simulink model "OMAP_ver_MIL10"  (R2018b)
settings: Solver=FixedStepDiscrete  StartTime=0.0  StopTime=10.0  FixedStep=0.01  RelTol=1e-3
undefined symbols (not defined in the file or in its folder): OMAP_Switch_EMS, OMAP_Switch_EPS, OMAP_Switch_ESC, OMAP_Switch_IC, OMAP_Switch_OTHER, TH_HMIClb_tiDgrdIconWarnHiDurT_C, TH_HMIClb_tiDgrdIconWarnLoDurT_C, TH_HMIClb_tiDgrdVocWarnDurT_C, TH_HMIClb_tiHndOffTxtWarnT_C, TH_HMIClb_tiHndOffVocWarnT_C, TH_HMIClb_tiSWALimFlgDetT_C, TH_HMIClb_tiTxtLimT_C
libraries: simulink x118
(part 7 of 9)

== system OMAP_ver_MIL10/OMAP_Module/ACCS_Direct/ACCS_Define/Human_Machine_Interface(ACC_HMI)/Text_PopUp/ACC_ON ==
  In1 : Inport
  In2 : Inport  Port=2
  ACCICA_Flag : Inport  Port=3
  Chart : Stateflow chart  TreatAsAtomicUnit=on
  Compare To Constant{1..2,6,9} (4 alike) : simulink/Logic and Bit Operations/Compare To Constant  relop===  const=1  OutDataTypeStr=boolean
  Compare To Constant10 : simulink/Logic and Bit Operations/Compare To Constant  relop=~=  const=1  OutDataTypeStr=boolean
  Compare To Constant11 : simulink/Logic and Bit Operations/Compare To Constant  relop=~=  const=15  OutDataTypeStr=boolean
  Compare To Constant14 : simulink/Logic and Bit Operations/Compare To Constant  relop===  const=3  OutDataTypeStr=boolean
  Compare To Constant3 : simulink/Logic and Bit Operations/Compare To Constant  relop===  const=2  OutDataTypeStr=boolean
  Compare To Constant4 : simulink/Logic and Bit Operations/Compare To Constant  relop=~=  const=1  OutDataTypeStr=boolean
  Compare To Constant5 : simulink/Logic and Bit Operations/Compare To Constant  relop=~=  const=0  OutDataTypeStr=boolean
  Compare To Constant7 : simulink/Logic and Bit Operations/Compare To Constant  relop===  const=0  OutDataTypeStr=boolean
  Compare To Constant8 : simulink/Logic and Bit Operations/Compare To Constant  relop===  const=0  OutDataTypeStr=boolean
  Logical Operator : Logic  Inputs=3  AllPortsSameDT=off  OutDataTypeStr=boolean
  Logical Operator1 : Logic  AllPortsSameDT=off  OutDataTypeStr=boolean
  Logical Operator2 : Logic  AllPortsSameDT=off  OutDataTypeStr=boolean
  Logical Operator3 : Logic  AllPortsSameDT=off  OutDataTypeStr=boolean
  Logical Operator4 : Logic  Operator=OR  AllPortsSameDT=off  OutDataTypeStr=boolean
  Logical Operator5 : Logic  Inputs=3  AllPortsSameDT=off  OutDataTypeStr=boolean
  Logical Operator9 : Logic  Operator=OR  AllPortsSameDT=off  OutDataTypeStr=boolean
  Unit Delay : UnitDelay  SampleTime=-1
  Unit Delay1 : UnitDelay  SampleTime=-1
  Unit Delay2 : UnitDelay  SampleTime=-1
  Out1 : Outport
  wires:
  Compare To Constant14/1 -> Logical Operator9/2
  Compare To Constant1/1 -> Logical Operator/1
  Logical Operator/1 -> Chart/1(data)
  Logical Operator9/1 -> Logical Operator/2
  Unit Delay/1 -> Compare To Constant1/1
  Compare To Constant3/1 -> Logical Operator9/1
  Chart/1(Value) -> Out1/1
  In2/1 -> Compare To Constant4/1, Unit Delay1/1
  Unit Delay1/1 -> Compare To Constant2/1
  Compare To Constant2/1 -> Logical Operator1/1
  Compare To Constant4/1 -> Logical Operator1/2
  Logical Operator4/1 -> Chart/2(data1)
  In1/1 -> Compare To Constant11/1, Compare To Constant10/1, Compare To Constant5/1, Compare To Constant14/1, Compare To Constant3/1, Unit Delay/1
  Logical Operator5/1 -> Logical Operator2/2
  ACCICA_Flag/1 -> Compare To Constant8/1, Compare To Constant9/1, Compare To Constant7/1, Unit Delay2/1
  Unit Delay2/1 -> Compare To Constant6/1
  Compare To Constant6/1 -> Logical Operator3/1
  Compare To Constant7/1 -> Logical Operator3/2
  Logical Operator3/1 -> Logical Operator2/1
  Logical Operator2/1 -> Chart/3(data2)
  Compare To Constant8/1 -> Logical Operator/3
  Logical Operator1/1 -> Logical Operator4/2
  Compare To Constant9/1 -> Logical Operator4/1
  Compare To Constant5/1 -> Logical Operator5/1
  Compare To Constant10/1 -> Logical Operator5/2
  Compare To Constant11/1 -> Logical Operator5/3

== system OMAP_ver_MIL10/OMAP_Module/ACCS_Direct/ACCS_Define/Human_Machine_Interface(ACC_HMI)/Text_PopUp/ACC_go_request ==
  In1 : Inport
  Compare To Constant1 : simulink/Logic and Bit Operations/Compare To Constant  relop===  const=1  OutDataTypeStr=boolean
  <GoRequest> : Outport
  wires:
  In1/1 -> Compare To Constant1/1
  Compare To Constant1/1 -> <GoRequest>/1

== system OMAP_ver_MIL10/OMAP_Module/ACCS_Direct/ACCS_Define/Human_Machine_Interface(ACC_HMI)/Text_PopUp/Please_Take_Over_the_Car ==
  In1 : Inport
  Chart1 : Stateflow chart  TreatAsAtomicUnit=on
  Compare To Constant1 : simulink/Logic and Bit Operations/Compare To Constant  relop===  const=6  OutDataTypeStr=boolean
  Compare To Constant18 : simulink/Logic and Bit Operations/Compare To Constant  relop===  const=6  OutDataTypeStr=boolean
  Compare To Constant19 : simulink/Logic and Bit Operations/Compare To Constant  relop===  const=4  OutDataTypeStr=boolean
  Compare To Constant2 : simulink/Logic and Bit Operations/Compare To Constant  relop=~=  const=6  OutDataTypeStr=boolean
  Logical Operator1 : Logic  AllPortsSameDT=off  OutDataTypeStr=boolean
  Logical Operator7 : Logic  AllPortsSameDT=off  OutDataTypeStr=boolean
  Unit Delay1 : UnitDelay  SampleTime=-1
  Unit Delay2 : UnitDelay  SampleTime=-1
  Out1 : Outport
  wires:
  Logical Operator7/1 -> Chart1/1(IN)
  Compare To Constant18/1 -> Logical Operator7/2
  Unit Delay2/1 -> Compare To Constant19/1
  Compare To Constant19/1 -> Logical Operator7/1
  Chart1/1(Value) -> Out1/1
  Unit Delay1/1 -> Compare To Constant1/1
  Compare To Constant1/1 -> Logical Operator1/1
  Compare To Constant2/1 -> Logical Operator1/2
  Logical Operator1/1 -> Chart1/2(OUT)
  In1/1 -> Unit Delay1/1, Compare To Constant2/1, Compare To Constant18/1, Unit Delay2/1

== system OMAP_ver_MIL10/OMAP_Module/ACCS_Direct/ACCS_Define/Human_Machine_Interface(ACC_HMI)/Text_PopUp/Please_Take_Over_the_Car_immediataly ==
  ESC_DecTar : Inport
  BRAKE_RELEASED_FAILSAFE1 : Constant  Value=0  OutDataTypeStr=boolean
  Chart1 : Stateflow chart  TreatAsAtomicUnit=on
  Out1 : Outport
  wires:
  Chart1/1(Value) -> Out1/1
  ESC_DecTar/1 -> Chart1/1(ESC_DecTar)
  BRAKE_RELEASED_FAILSAFE1/1 -> Chart1/2(BRAKE_RELEASED_FAILSAFE)

== system OMAP_ver_MIL10/OMAP_Module/ICA_Direct_G59/ICA_Define/Subsystem1/Dspl/DsplPrcs ==
  DsplPrcs_stStWhlHld : Inport
  DsplPrcs_stTkOvStChk : Inport  Port=2
  DsplPrcs_facmL0Ql : Inport  Port=3
  DsplPrcs_facmR0Ql : Inport  Port=4
  DsplPrcs_facmL0Type : Inport  Port=5
  DsplPrcs_facmR0Type : Inport  Port=6
  DsplPrcs_stTHState : Inport  Port=7
  DsplPrcs_bsFromFMCMsg : Inport  Port=8
  DsplPrcs_stTHFKeyState : Inport  Port=9
  DsplPrcs_stVehSty : Inport  Port=10
  DsplPrcs_tfAddVocCmd : Inport  Port=11
  DsplPrcs_stSWALimFlg : Inport  Port=12
  DsplPrcs_dHndOffTxtWarnnum : Inport  Port=13
  DsplPrcs_dDgrdVocWarnDurnum : Inport  Port=14
  DsplPrcs_dHndOffVocWarnnum : Inport  Port=15
  DsplPrcs_dTxtLimnum : Inport  Port=16
  DsplPrcs_dDgrdIconWarnHiDurnum : Inport  Port=17
  DsplPrcs_dDgrdIconWarnLoDurnum : Inport  Port=18
  DsplPrcs_tiSWALimFlgDetnum : Inport  Port=19
  DsplPrcs_dDgrdIconWarnflag : Inport  Port=20
  Bus Creator1 : BusCreator  Inputs=4
  Bus Selector : BusSelector  OutputSignals=stLaneDspl,stL0DispType,stR0DispType
  Bus Selector1 : BusSelector  OutputSignals=ACC_State
  Data Type Conversion1 : DataTypeConversion  OutDataTypeStr=uint16
  Icon : Subsystem
  Lane : Subsystem
  Lane_old : Subsystem
  Manual Switch : ManualSwitch
  Txt : Subsystem
  Voc : Subsystem
  DsplPrcs_stTxtDspl : Outport
  DsplPrcs_stIconDspl : Outport  Port=2
  DsplPrcs_stLaneDspl : Outport  Port=3
  DsplPrcs_stL0DispType : Outport  Port=4
  DsplPrcs_stR0DispType : Outport  Port=5
  DsplPrcs_stVocDspl : Outport  Port=6
  DsplPrcs_bsMon : Outport  Port=7
  wires:
  DsplPrcs_stTHFKeyState/1 -> Txt/4(Txt_stTHFKeyState)
  Txt/1(Txt_stTxtDspl) -> DsplPrcs_stTxtDspl/1
  DsplPrcs_stTHState/1 -> Txt/6(Txt_stTHState), Lane_old/1(Lane_stTHState), Voc/2(Voc_stTHState), Lane/1(Lane_stTHState), Icon/1(Icon_stTHState)
  Icon/1(Icon_stIconDspl) -> Bus Creator1/2, DsplPrcs_stIconDspl/1  "ICA_status_icon"
  Lane/1(Lane_stLaneDspl) -> Bus Creator1/3, Bus Selector/1  "Vehicle_Lane_Display"
  Txt/2(Txt_bsMon) -> Bus Creator1/1  "ICA_HMI_Txt_Mon"
  Bus Creator1/1 -> DsplPrcs_bsMon/1
  DsplPrcs_stStWhlHld/1 -> Voc/1(Voc_stStWhlHld), Txt/1(Txt_stStWhlHld)
  DsplPrcs_dHndOffTxtWarnnum/1 -> Txt/5(Txt_dHndOffTxtWarnnum)
  Voc/1(Voc_stVocDspl) -> DsplPrcs_stVocDspl/1, Bus Creator1/4  "Hands_off_warning"
  DsplPrcs_dHndOffVocWarnnum/1 -> Voc/4(Voc_dHndOffVocWarnnum)
  DsplPrcs_dDgrdVocWarnDurnum/1 -> Voc/3(Voc_dDgrdVocWarnDurnum)
  DsplPrcs_bsFromFMCMsg/1 -> Txt/3(Txt_bsFromFMCMsg), Bus Selector1/1
  Data Type Conversion1/1 -> Icon/2(Icon_stACCState)
  Bus Selector1/1 -> Data Type Conversion1/1  "<ACC_State>"
  DsplPrcs_dTxtLimnum/1 -> Txt/7(Txt_dTxtLimnum)
  DsplPrcs_facmL0Ql/1 -> Lane_old/3(Lane_facmL0Ql), Lane/3(Lane_facmL0Ql)
  DsplPrcs_facmR0Ql/1 -> Lane_old/4(Lane_facmR0Ql), Lane/4(Lane_facmR0Ql)
  DsplPrcs_stVehSty/1 -> Lane/2(Lane_stVehSty), Lane_old/2(Lane_stVehSty), Voc/5(Voc_stVehSty), Txt/2(Txt_stVehSty)
  DsplPrcs_tfAddVocCmd/1 -> Voc/6(Voc_tfAddVocCmd)
  DsplPrcs_dDgrdIconWarnHiDurnum/1 -> Icon/3(Icon_dDgrdIconWarnHiDurnum)
  DsplPrcs_dDgrdIconWarnLoDurnum/1 -> Icon/4(Icon_dDgrdIconWarnLoDurnum)
  DsplPrcs_dDgrdIconWarnflag/1 -> Icon/5(Icon_dDgrdIconWarnflag)
  DsplPrcs_stSWALimFlg/1 -> Txt/8(Txt_stSWALimFlg)
  DsplPrcs_tiSWALimFlgDetnum/1 -> Txt/9(Txt_tiSWALimFlgDetnum)
  DsplPrcs_stTkOvStChk/1 -> Txt/10(Txt_stTkOvStChk)
  DsplPrcs_facmL0Type/1 -> Lane/5(Lane_facmL0Type)
  DsplPrcs_facmR0Type/1 -> Lane/6(Lane_facmR0Type)
  Bus Selector/1 -> Manual Switch/1  "<stLaneDspl>"
  Bus Selector/2 -> DsplPrcs_stL0DispType/1  "<stL0DispType>"
  Bus Selector/3 -> DsplPrcs_stR0DispType/1  "<stR0DispType>"
  Lane_old/1(Lane_stLaneDspl) -> Manual Switch/2
  Manual Switch/1 -> DsplPrcs_stLaneDspl/1

== system OMAP_ver_MIL10/OMAP_Module/ICA_Direct_G59/ICA_Define/Subsystem1/Dspl/TimePrcs ==
  TimePrcs_tiHndOffTxtWarnT_C : Inport
  TimePrcs_tiDgrdVocWarnDurT_C : Inport  Port=2
  TimePrcs_tiHndOffVocWarnT_C : Inport  Port=3
  TimePrcs_tiTxtLimT_C : Inport  Port=4
  TimePrcs_tiDgrdIconWarnHiDurT_C : Inport  Port=5
  TimePrcs_tiDgrdIconWarnLoDurT_C : Inport  Port=6
  TimePrcs_tiSWALimFlgDetT_C : Inport  Port=7
  TimePrcs_tiCalcPer_C : Inport  Port=8
  Divide{,1..6} (7 alike) : Product  Inputs=*/  OutDataTypeStr=uint16
  Switch : Switch  Criteria=u2 ~= 0  OutDataTypeStr=single
  constant : Constant  Value=0.01  OutDataTypeStr=single
  TimePrcs_dHndOffTxtWarnnum : Outport
  TimePrcs_dDgrdVocWarnDurnum : Outport  Port=2
  TimePrcs_dHndOffVocWarnnum : Outport  Port=3
  TimePrcs_dTxtLimnum : Outport  Port=4
  TimePrcs_dDgrdIconWarnHiDurnum : Outport  Port=5
  TimePrcs_dDgrdIconWarnLoDurnum : Outport  Port=6
  TimePrcs_tiSWALimFlgDetnum : Outport  Port=7
  wires:
  Divide/1 -> TimePrcs_dHndOffTxtWarnnum/1
  TimePrcs_tiCalcPer_C/1 -> Switch/1, Switch/2
  constant/1 -> Switch/3
  TimePrcs_tiHndOffTxtWarnT_C/1 -> Divide/1
  Switch/1 -> Divide5/2, Divide4/2, Divide3/2, Divide2/2, Divide1/2, Divide/2, Divide6/2
  TimePrcs_tiDgrdVocWarnDurT_C/1 -> Divide1/1
  TimePrcs_tiHndOffVocWarnT_C/1 -> Divide2/1
  TimePrcs_tiTxtLimT_C/1 -> Divide3/1
  Divide1/1 -> TimePrcs_dDgrdVocWarnDurnum/1
  Divide2/1 -> TimePrcs_dHndOffVocWarnnum/1
  Divide3/1 -> TimePrcs_dTxtLimnum/1
  TimePrcs_tiDgrdIconWarnHiDurT_C/1 -> Divide4/1
  Divide4/1 -> TimePrcs_dDgrdIconWarnHiDurnum/1
  TimePrcs_tiDgrdIconWarnLoDurT_C/1 -> Divide5/1
  Divide5/1 -> TimePrcs_dDgrdIconWarnLoDurnum/1
  Divide6/1 -> TimePrcs_tiSWALimFlgDetnum/1
  TimePrcs_tiSWALimFlgDetT_C/1 -> Divide6/1

== system OMAP_ver_MIL10/OMAP_Module/ICA_Direct_G59/ICA_Define/Subsystem1/Subsystem/Subsystem ==
  HiDurnum : Inport
  LoDurnum : Inport  Port=2
  Add : Sum
  Constant1 : Constant  Value=0  OutDataTypeStr=uint16
  Constant8 : Constant  OutDataTypeStr=uint16
  Count : Terminator
  Relational Operator1 : RelationalOperator  Operator=<=  OutDataTypeStr=boolean  RndMeth=Nearest
  Relational Operator2 : RelationalOperator  Operator=<=  OutDataTypeStr=boolean  RndMeth=Nearest
  Sum : Sum  OutDataTypeStr=Inherit: Inherit via back propagation  InputSameDT=on
  Unit Delay1 : UnitDelay  SampleTime=-1
  Unit Delay2 : UnitDelay  SampleTime=-1
  reset switch1 : Switch  Criteria=u2 ~= 0  Threshold=1  OutDataTypeStr=Inherit: Inherit via back propagation  InputSameDT=on
  Signal : Outport
  wires:
  Unit Delay2/1 -> Sum/2
  HiDurnum/1 -> Relational Operator2/2, Add/1
  Unit Delay1/1 -> [reset]
  Add/1 -> Relational Operator1/1
  [reset] -> reset switch1/2
  Constant8/1 -> Sum/1
  Relational Operator1/1 -> Unit Delay1/1
  reset switch1/1 -> Count/1, Relational Operator2/1, Relational Operator1/2, Unit Delay2/1
  Constant1/1 -> reset switch1/1
  LoDurnum/1 -> Add/2
  Relational Operator2/1 -> Signal/1
  Sum/1 -> reset switch1/3

== system OMAP_ver_MIL10/OMAP_Module/ICA_Direct_G59/ICA_Define/Subsystem1/Dspl/DsplPrcs/Icon ==
  Icon_stTHState : Inport
  Icon_stACCState : Inport  Port=2
  Icon_dDgrdIconWarnHiDurnum : Inport  Port=3
  Icon_dDgrdIconWarnLoDurnum : Inport  Port=4
  Icon_dDgrdIconWarnflag : Inport  Port=5
  Constant : Constant  Value=0  OutDataTypeStr=uint16
  Constant1 : Constant  OutDataTypeStr=uint16
  Constant2 : Constant  Value=2  OutDataTypeStr=uint16
  Constant3 : Constant  Value=3  OutDataTypeStr=uint16
  Constant4 : Constant  Value=0  OutDataTypeStr=uint16
  Constant5 : Constant  Value=4  OutDataTypeStr=uint16
  Constant6 : Constant  OutDataTypeStr=boolean
  FaultInhib : Subsystem
  If : If  NumInputs=2  IfExpression=u1==0  ElseIfExpressions=u1==1|u1==2|u1==6|u1==7|u1==8,u1==3,u1==4,u1==5&u2==1,u1==5&u2==0
  If1 : If  IfExpression=u1 == 0
  Merge : Merge  Inputs=7
  Merge1 : Merge
  OragneIcon : Scope  NumInputPorts=6
  Unit Delay : UnitDelay  SampleTime=-1
  Unit Delay1 : UnitDelay  SampleTime=-1
  else : Subsystem  TreatAsAtomicUnit=on
  gray : Subsystem  TreatAsAtomicUnit=on
  green : Subsystem  TreatAsAtomicUnit=on
  hold_last : Subsystem  TreatAsAtomicUnit=on
  if : Subsystem  TreatAsAtomicUnit=on
  off : Subsystem  TreatAsAtomicUnit=on
  off_fault : Subsystem  TreatAsAtomicUnit=on
  orange : Subsystem  TreatAsAtomicUnit=on
  red : Subsystem  TreatAsAtomicUnit=on
  Icon_stIconDspl : Outport
  wires:
  Icon_stTHState/1 -> FaultInhib/1(FaultInhib_stTHState), If/1, Unit Delay/1
  Icon_stACCState/1 -> FaultInhib/3(FaultInhib_stACCState)
  Unit Delay/1 -> FaultInhib/2(FaultInhib_stLstTHState)
  If/4 -> orange/Action
  If/2 -> gray/Action
  If/1 -> off/Action
  If/7 -> hold_last/Action
  If/3 -> green/Action
  FaultInhib/1(FaultInhib_stFaultInhibFlg) -> If/2
  If/5 -> off_fault/Action
  If/6 -> red/Action
  orange/1(Out1) -> Merge/4
  Merge/1 -> Unit Delay1/1, OragneIcon/1, Icon_stIconDspl/1  "Icon_stIconDspl"
  Unit Delay1/1 -> hold_last/1(In1)
  off/1(Out1) -> Merge/1
  gray/1(Out1) -> Merge/2
  green/1(Out1) -> Merge/3
  off_fault/1(Out1) -> Merge/5
  red/1(Out1) -> Merge/6
  hold_last/1(Out1) -> Merge/7
  Constant/1 -> off/1(In1)
  Constant5/1 -> red/1(In1)
  Constant4/1 -> off_fault/1(In1)
  Constant3/1 -> orange/1(In1)
  Constant1/1 -> gray/1(In1)
  Constant2/1 -> green/1(In1)
  If1/1 -> if/Action
  If1/2 -> else/Action
  Constant6/1 -> if/1(In1)
  if/1(Out1) -> Merge1/1
  Merge1/1 -> OragneIcon/2, orange/2(In2)  "orange_enable"
  else/2(counter_status) -> Merge1/2
  Icon_dDgrdIconWarnflag/1 -> OragneIcon/4, If1/1  "DgrdIconWarnflag"
  Icon_dDgrdIconWarnHiDurnum/1 -> OragneIcon/5, else/1(HiDurnum)  "DgrdIconWarnHinum"
  Icon_dDgrdIconWarnLoDurnum/1 -> else/2(LoDurnum), OragneIcon/6  "DgrdIconWarnLonum"
  else/1(count) -> OragneIcon/3  "DgrdIcon_count"

== system OMAP_ver_MIL10/OMAP_Module/ICA_Direct_G59/ICA_Define/Subsystem1/Dspl/DsplPrcs/Lane ==
  note: ->0
  note: ->1
  note: ->2
  note: ->14
  note: ->15
  note: ->16
  Lane_stTHState : Inport
  Lane_stVehSty : Inport  Port=2
  Lane_facmL0Ql : Inport  Port=3
  Lane_facmR0Ql : Inport  Port=4
  Lane_facmL0Type : Inport  Port=5
  Lane_facmR0Type : Inport  Port=6
  Bus Creator : BusCreator  Inputs=3
  Compare To Constant3 : simulink/Logic and Bit Operations/Compare To Constant  relop===  const=uint16(3)  OutDataTypeStr=boolean
  Compare To Constant4 : simulink/Logic and Bit Operations/Compare To Constant  relop===  const=uint16(3)  OutDataTypeStr=boolean
  Compare To Zero : simulink/Logic and Bit Operations/Compare To Zero  relop===  OutDataTypeStr=boolean
  Constant1 : Constant  Value=14  OutDataTypeStr=uint16
  Constant10 : Constant  OutDataTypeStr=uint16
  Constant2 : Constant  Value=0  OutDataTypeStr=uint16
  Constant4 : Constant  Value=2  OutDataTypeStr=uint16
  Constant5 : Constant  Value=0  OutDataTypeStr=uint16
  Constant6 : Constant  OutDataTypeStr=uint16
  Constant7 : Constant  Value=3  OutDataTypeStr=uint16
  Constant8 : Constant  OutDataTypeStr=uint16
  Constant9 : Constant  Value=3  OutDataTypeStr=uint16
  Data Type Conversion{,1,3..5} (5 alike) : DataTypeConversion  OutDataTypeStr=uint16
  If : If  NumInputs=3  IfExpression=u1==0|u1==5  ElseIfExpressions=(u1==1|u1==2|u1==4|u1==6|u1==7|u1==8)&(u2<3&u3<3),(u1==1|u1==2|u1==4|u1==6|u1==7|u1==8)&(u2==3&u3==3),u1==3,u1==98,u1==99
  Merge : Merge  Inputs=5
  Merge1 : Merge  Inputs=5
  Merge2 : Merge  Inputs=5
  Subsystem : Subsystem
  Switch : Switch  Criteria=u2 ~= 0
  Switch1 : Switch  Criteria=u2 ~= 0
  Switch2 : Switch  Criteria=u2 ~= 0
  Terminator : Terminator
  Terminator1 : Terminator
  left_no_right_no : Subsystem  TreatAsAtomicUnit=on
  left_no_right_no1 : Subsystem  TreatAsAtomicUnit=on
  left_no_right_ok : Subsystem  TreatAsAtomicUnit=on
  left_ok_right_no : Subsystem  TreatAsAtomicUnit=on
  left_ok_right_ok : Subsystem  TreatAsAtomicUnit=on
  Lane_stLaneDspl : Outport
  wires:
  Lane_stTHState/1 -> Data Type Conversion3/1
  Data Type Conversion3/1 -> If/1
  Bus Creator/1 -> Subsystem/1(In1), Switch/1
  Lane_facmL0Ql/1 -> If/2
  Lane_facmR0Ql/1 -> If/3
  Lane_stVehSty/1 -> Data Type Conversion1/1
  Compare To Zero/1 -> Subsystem/Enable, Switch/2
  Switch/1 -> Lane_stLaneDspl/1
  Data Type Conversion1/1 -> Compare To Zero/1
  Subsystem/1(Out1) -> Switch/3
  Constant5/1 -> left_no_right_no/1(In1)
  Lane_facmL0Type/1 -> Compare To Constant3/1
  Compare To Constant3/1 -> Switch1/2
  Constant7/1 -> Switch1/1
  Constant8/1 -> Switch1/3
  Switch1/1 -> [stL0DispType]
  Lane_facmR0Type/1 -> Compare To Constant4/1
  Compare To Constant4/1 -> Switch2/2
  Constant9/1 -> Switch2/1
  Constant10/1 -> Switch2/3
  Switch2/1 -> [stR0DispType]
  [stL0DispType] -> left_ok_right_ok/2(In2)
  [stR0DispType] -> left_ok_right_ok/3(In3)
  Constant4/1 -> left_ok_right_ok/1(In1)
  If/1 -> left_no_right_no/Action
  If/2 -> left_ok_right_ok/Action
  If/3 -> left_ok_right_no/Action
  If/4 -> left_no_right_ok/Action
  If/7 -> left_no_right_no1/Action
  left_no_right_no/1(Out1) -> Merge/1
  left_ok_right_ok/1(Out1) -> Merge/2
  left_ok_right_no/1(Out1) -> Merge/3
  left_no_right_ok/1(Out1) -> Merge/4
  left_no_right_no1/1(Out1) -> Merge/5
  left_no_right_no/2(Out2) -> Merge1/1
  left_ok_right_ok/2(Out2) -> Merge1/2
  left_ok_right_no/2(Out2) -> Merge1/3
  left_no_right_ok/2(Out2) -> Merge1/4
  left_no_right_no1/2(Out2) -> Merge1/5
  left_no_right_no/3(Out3) -> Merge2/1
  left_ok_right_ok/3(Out3) -> Merge2/2
  left_ok_right_no/3(Out3) -> Merge2/3
  left_no_right_ok/3(Out3) -> Merge2/4
  left_no_right_no1/3(Out3) -> Merge2/5
  Merge/1 -> Data Type Conversion/1
  Merge1/1 -> Data Type Conversion4/1
  Merge2/1 -> Data Type Conversion5/1
  Data Type Conversion/1 -> Bus Creator/1  "stLaneDspl"
  Data Type Conversion4/1 -> Bus Creator/2  "stL0DispType"
  Data Type Conversion5/1 -> Bus Creator/3  "stR0DispType"
  [stR0DispType] -> left_no_right_no/3(In3)
  [stL0DispType] -> left_no_right_no/2(In2)
  Constant6/1 -> left_ok_right_no/1(In1)
  [stR0DispType] -> left_ok_right_no/3(In3)
  [stL0DispType] -> left_ok_right_no/2(In2)
  [stL0DispType] -> left_no_right_ok/2(In2)
  [stR0DispType] -> left_no_right_ok/3(In3)
  Constant1/1 -> left_no_right_ok/1(In1)
  Constant2/1 -> left_no_right_no1/1(In1)
  [stR0DispType] -> left_no_right_no1/3(In3)
  [stL0DispType] -> left_no_right_no1/2(In2)
  If/5 -> Terminator/1
  If/6 -> Terminator1/1

== system OMAP_ver_MIL10/OMAP_Module/ICA_Direct_G59/ICA_Define/Subsystem1/Dspl/DsplPrcs/Lane_old ==
  Lane_stTHState : Inport
  Lane_stVehSty : Inport  Port=2
  Lane_facmL0Ql : Inport  Port=3
  Lane_facmR0Ql : Inport  Port=4
  Compare To Constant : simulink/Logic and Bit Operations/Compare To Constant  relop===  const=uint16(0)  OutDataTypeStr=boolean
  Compare To Constant1 : simulink/Logic and Bit Operations/Compare To Constant  relop===  const=uint16(5)  OutDataTypeStr=boolean
  Compare To Constant2 : simulink/Logic and Bit Operations/Compare To Constant  relop===  const=uint16(1)  OutDataTypeStr=boolean
  Compare To Zero : simulink/Logic and Bit Operations/Compare To Zero  relop===  OutDataTypeStr=boolean
  Constant : Constant  Value=0  OutDataTypeStr=uint16
  Constant1 : Constant  Value=2  OutDataTypeStr=uint16
  Constant2 : Constant  Value=5  OutDataTypeStr=uint16
  Constant3 : Constant  Value=3  OutDataTypeStr=uint16
  Constant4 : Constant  Value=4  OutDataTypeStr=uint16
  Data Type Conversion1 : DataTypeConversion  OutDataTypeStr=uint16
  Data Type Conversion2 : DataTypeConversion  OutDataTypeStr=uint16
  Data Type Conversion3 : DataTypeConversion  OutDataTypeStr=uint16
  If : If  NumInputs=3  IfExpression=u1 == 1  ElseIfExpressions=u2 < 3 & u3 < 3,u2 == 3 & u3 == 3,u2 == 3 & u3 < 3
  Logical Operator : Logic  Operator=OR  AllPortsSameDT=off  OutDataTypeStr=boolean
  Merge : Merge  Inputs=5
  Subsystem : Subsystem
  Switch : Switch  Criteria=u2 ~= 0
  both_gray : Subsystem  TreatAsAtomicUnit=on
  both_green : Subsystem  TreatAsAtomicUnit=on
  left_green : Subsystem  TreatAsAtomicUnit=on
  no_lane : Subsystem  TreatAsAtomicUnit=on
  right_green : Subsystem  TreatAsAtomicUnit=on
  Lane_stLaneDspl : Outport
  wires:
  Data Type Conversion2/1 -> Switch/3
  Data Type Conversion1/1 -> Compare To Zero/1
  Switch/1 -> Lane_stLaneDspl/1
  Subsystem/1(Out1) -> Data Type Conversion2/1
  Compare To Zero/1 -> Switch/2, Subsystem/Enable
  Lane_stVehSty/1 -> Data Type Conversion1/1
  Constant4/1 -> right_green/1(In1)
  Constant3/1 -> left_green/1(In1)
  Constant2/1 -> both_green/1(In1)
  Constant1/1 -> both_gray/1(In1)
  Constant/1 -> no_lane/1(In1)
  right_green/1(Out1) -> Merge/5
  left_green/1(Out1) -> Merge/4
  both_green/1(Out1) -> Merge/3
  both_gray/1(Out1) -> Merge/2
  no_lane/1(Out1) -> Merge/1
  If/5 -> right_green/Action
  If/4 -> left_green/Action
  If/3 -> both_green/Action
  If/2 -> both_gray/Action
  Lane_facmR0Ql/1 -> If/3
  Lane_facmL0Ql/1 -> If/2
  Merge/1 -> Switch/1, Subsystem/1(In1)
  If/1 -> no_lane/Action
  Data Type Conversion3/1 -> If/1
  Compare To Constant2/1 -> Data Type Conversion3/1
  Logical Operator/1 -> Compare To Constant2/1
  Compare To Constant1/1 -> Logical Operator/2
  Compare To Constant/1 -> Logical Operator/1
  Lane_stTHState/1 -> Compare To Constant1/1, Compare To Constant/1

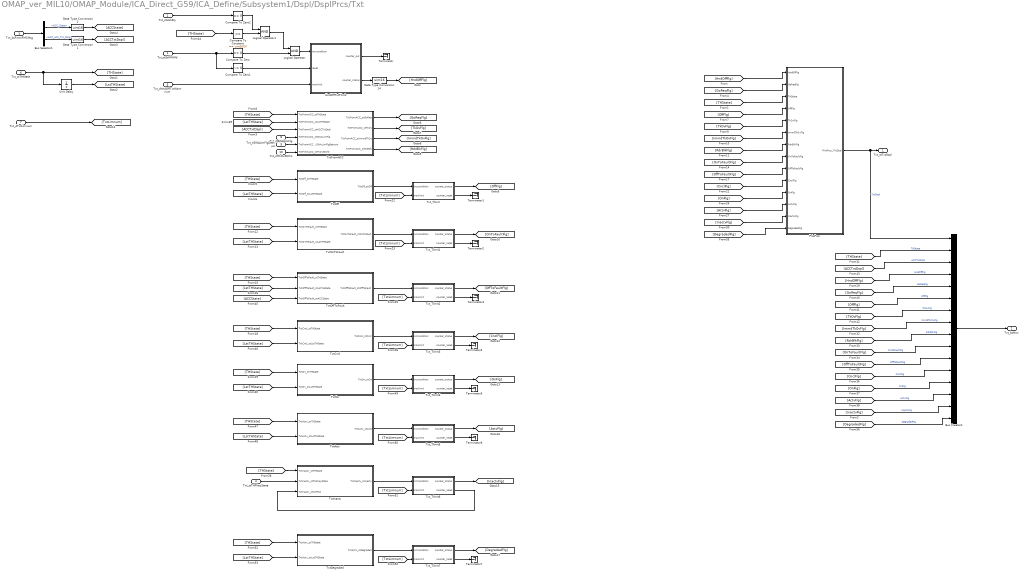
== system OMAP_ver_MIL10/OMAP_Module/ICA_Direct_G59/ICA_Define/Subsystem1/Dspl/DsplPrcs/Txt ==
  Txt_stStWhlHld : Inport
  Txt_stVehSty : Inport  Port=2
  Txt_bsFromFMCMsg : Inport  Port=3
  Txt_stTHFKeyState : Inport  Port=4
  Txt_dHndOffTxtWarnnum : Inport  Port=5
  Txt_stTHState : Inport  Port=6
  Txt_dTxtLimnum : Inport  Port=7
  Txt_stSWALimFlg : Inport  Port=8
  Txt_tiSWALimFlgDetnum : Inport  Port=9
  Txt_stTkOvStChk : Inport  Port=10
  Bus Creator1 : BusCreator  Inputs=16
  Bus Selector1 : BusSelector  OutputSignals=ACC_State,ACC_HMI_Txt_Disp
  Compare To Constant : simulink/Logic and Bit Operations/Compare To Constant  relop===  const=uint16(3)  OutDataTypeStr=boolean
  Compare To Zero : simulink/Logic and Bit Operations/Compare To Zero  relop===  OutDataTypeStr=boolean
  Compare To Zero1 : simulink/Logic and Bit Operations/Compare To Zero  relop=~=  OutDataTypeStr=boolean
  Compare To Zero2 : simulink/Logic and Bit Operations/Compare To Zero  relop===  OutDataTypeStr=boolean
  Data Type Conversion1 : DataTypeConversion  OutDataTypeStr=uint16
  Data Type Conversion14 : DataTypeConversion  OutDataTypeStr=uint16
  Data Type Conversion2 : DataTypeConversion  OutDataTypeStr=uint16
  HndOffTxtTlimit : Subsystem
  Logical Operator : Logic  AllPortsSameDT=off  OutDataTypeStr=boolean
  Logical Operator1 : Logic  AllPortsSameDT=off  OutDataTypeStr=boolean
  PrioPrcs : MATLAB Function  TreatAsAtomicUnit=on
  Terminator{,1..7} (8 alike) : Terminator
  TxtActv : Subsystem
  TxtCncl : Subsystem
  TxtDegraded : Subsystem
  TxtFromACC : Subsystem
  TxtInactv : Subsystem
  TxtOff : Subsystem
  TxtOffToFault : Subsystem
  TxtOn : Subsystem
  TxtOnToFault : Subsystem
  Txt_Tlimit : Subsystem
  Txt_Tlimit1 : Subsystem
  Txt_Tlimit2 : Subsystem
  Txt_Tlimit3 : Subsystem
  Txt_Tlimit4 : Subsystem
  Txt_Tlimit5 : Subsystem
  Txt_Tlimit6 : Subsystem
  Txt_Tlimit7 : Subsystem
  Unit Delay : UnitDelay  SampleTime=-1
  Txt_stTxtDspl : Outport
  Txt_bsMon : Outport  Port=2
  wires:
  Compare To Zero/1 -> Logical Operator/2
  Txt_dHndOffTxtWarnnum/1 -> HndOffTxtTlimit/3(maxlimit)
  Compare To Zero1/1 -> HndOffTxtTlimit/2(reset)
  HndOffTxtTlimit/1(counter_out) -> Terminator/1
  Txt_stStWhlHld/1 -> Compare To Zero1/1, Compare To Zero/1
  HndOffTxtTlimit/2(counter_status) -> Data Type Conversion14/1
  [HndOffFlg] -> PrioPrcs/1(HndOffFlg)
  Txt_stTHState/1 -> Unit Delay/1, [THState]
  Unit Delay/1 -> [LstTHState]
  [THState] -> PrioPrcs/3(THState)
  [OffFlg] -> PrioPrcs/4(OffFlg)
  PrioPrcs/1(PrioPrcs_TxtDspl) -> Bus Creator1/1, Txt_stTxtDspl/1  "TxtDspl"
  [GoReqFlg] -> PrioPrcs/2(GoReqFlg)
  [TkOvFlg] -> PrioPrcs/5(TkOvFlg)
  [ImmdTkOvFlg] -> PrioPrcs/6(ImmdTkOvFlg)
  [RdrBlkFlg] -> PrioPrcs/7(RdrBlkFlg)
  [OnToFaultFlg] -> PrioPrcs/8(OnToFaultFlg)
  [OffToFaultFlg] -> PrioPrcs/9(OffToFaultFlg)
  [CnclFlg] -> PrioPrcs/10(CnclFlg)
  [OnFlg] -> PrioPrcs/11(OnFlg)
  [ActvFlg] -> PrioPrcs/12(ActvFlg)
  [InactvFlg] -> PrioPrcs/13(InactvFlg)
  [THState] -> Bus Creator1/2  "THState"
  [ACCTxtDspl] -> Bus Creator1/3  "ACCTxtDspl"
  [HndOffFlg] -> Bus Creator1/4  "HndOffFlg"
  [GoReqFlg] -> Bus Creator1/5  "GoReqFlg"
  [OffFlg] -> Bus Creator1/6  "OffFlg"
  [TkOvFlg] -> Bus Creator1/7  "TkOvFlg"
  [ImmdTkOvFlg] -> Bus Creator1/8  "ImmdTkOvFlg"
  [RdrBlkFlg] -> Bus Creator1/9  "RdrBlkFlg"
  [OnToFaultFlg] -> Bus Creator1/10  "OnToFaultFlg"
  [OffToFaultFlg] -> Bus Creator1/11  "OffToFaultFlg"
  [CnclFlg] -> Bus Creator1/12  "CnclFlg"
  [OnFlg] -> Bus Creator1/13  "OnFlg"
  [ActvFlg] -> Bus Creator1/14  "ActvFlg"
  [InactvFlg] -> Bus Creator1/15  "InactvFlg"
  Bus Creator1/1 -> Txt_bsMon/1
  Data Type Conversion14/1 -> [HndOffFlg]
  [THState] -> Compare To Constant/1
  Compare To Constant/1 -> Logical Operator1/2
  Logical Operator/1 -> HndOffTxtTlimit/1(incrcondition)
  Txt_bsFromFMCMsg/1 -> Bus Selector1/1
  Data Type Conversion1/1 -> [ACCTxtDspl]
  Bus Selector1/2 -> Data Type Conversion1/1  "<ACC_HMI_Txt_Disp>"
  Data Type Conversion2/1 -> [ACCState]
  Bus Selector1/1 -> Data Type Conversion2/1  "<ACC_State>"
  [THState] -> TxtOffToFault/1(TxtOffToFault_stTHState)
  [LstTHState] -> TxtOffToFault/2(TxtOffToFault_stLstTHState)
  [ACCState] -> TxtOffToFault/3(TxtOffToFault_stACCState)
  [LstTHState] -> TxtOnToFault/2(TxtOnToFault_stLstTHState)
  [THState] -> TxtOnToFault/1(TxtOnToFault_stTHState)
  [THState] -> TxtCncl/1(TxtCncl_stTHState)
  [LstTHState] -> TxtCncl/2(TxtCncl_stLstTHState)
  [LstTHState] -> TxtOn/2(TxtOn_stLstTHState)
  [THState] -> TxtOn/1(TxtOn_stTHState)
  [LstTHState] -> TxtActv/2(TxtActv_stLstTHState)
  [THState] -> TxtActv/1(TxtActv_stTHState)
  [THState] -> TxtInactv/1(TxtInactv_stTHState)
  Txt_stTHFKeyState/1 -> TxtInactv/2(TxtInactv_stTHFKeyState)
  [LstTHState] -> TxtOff/2(TxtOff_stLstTHState)
  [THState] -> TxtOff/1(TxtOff_stTHState)
  [THState] -> TxtFromACC/1(TxtFromACC_stTHState)
  [LstTHState] -> TxtFromACC/2(TxtFromACC_stLstTHState)
  [ACCTxtDspl] -> TxtFromACC/3(TxtFromACC_stACCTxtDspl)
  TxtFromACC/1(TxtFromACC_stGoReq) -> [GoReqFlg]
  TxtFromACC/2(TxtFromACC_stTkOv) -> [TkOvFlg]
  TxtFromACC/3(TxtFromACC_stImmdTkOv) -> [ImmdTkOvFlg]
  TxtFromACC/4(TxtFromACC_stRdrBlk) -> [RdrBlkFlg]
  Txt_dTxtLimnum/1 -> [TxtLimnum]
  [TxtLimnum] -> Txt_Tlimit/2(maxlimit)
  TxtOff/1(TxtOff_stOff) -> Txt_Tlimit/1(incrcondition)
  Txt_Tlimit/1(counter_status) -> [OffFlg]
  Txt_Tlimit1/1(counter_status) -> [OnToFaultFlg]
  TxtOnToFault/1(TxtOnToFault_stOnToFault) -> Txt_Tlimit1/1(incrcondition)
  [TxtLimnum] -> Txt_Tlimit1/2(maxlimit)
  [TxtLimnum] -> Txt_Tlimit2/2(maxlimit)
  TxtOffToFault/1(TxtOffToFault_stOffToFault) -> Txt_Tlimit2/1(incrcondition)
  Txt_Tlimit2/1(counter_status) -> [OffToFaultFlg]
  Txt_Tlimit3/1(counter_status) -> [CnclFlg]
  TxtCncl/1(TxtCncl_stCncl) -> Txt_Tlimit3/1(incrcondition)
  [TxtLimnum] -> Txt_Tlimit3/2(maxlimit)
  [TxtLimnum] -> Txt_Tlimit4/2(maxlimit)
  TxtOn/1(TxtOn_stOn) -> Txt_Tlimit4/1(incrcondition)
  Txt_Tlimit4/1(counter_status) -> [OnFlg]
  Txt_Tlimit5/1(counter_status) -> [ActvFlg]
  TxtActv/1(TxtActv_stActv) -> Txt_Tlimit5/1(incrcondition)
  [TxtLimnum] -> Txt_Tlimit5/2(maxlimit)
  [TxtLimnum] -> Txt_Tlimit6/2(maxlimit)
  TxtInactv/1(TxtInactv_stInactv) -> Txt_Tlimit6/1(incrcondition)
  Txt_Tlimit6/1(counter_status) -> [InactvFlg]
  Txt_Tlimit6/2(counter_reset) -> TxtInactv/3(TxtInactv_stCntRst)
  Txt_Tlimit/2(counter_reset) -> Terminator1/1
  Txt_Tlimit1/2(counter_reset) -> Terminator2/1
  Txt_Tlimit2/2(counter_reset) -> Terminator3/1
  Txt_Tlimit3/2(counter_reset) -> Terminator4/1
  Txt_Tlimit4/2(counter_reset) -> Terminator5/1
  Txt_Tlimit5/2(counter_reset) -> Terminator6/1
  Txt_stSWALimFlg/1 -> TxtFromACC/4(TxtFromACC_stSWALimFlg)
  Txt_tiSWALimFlgDetnum/1 -> TxtFromACC/5(TxtFromACC_tiSWALimFlgDetnum)
  Txt_stTkOvStChk/1 -> TxtFromACC/6(TxtFromACC_stTkOvStChk)
  Txt_stVehSty/1 -> Compare To Zero2/1
  Compare To Zero2/1 -> Logical Operator1/1
  Logical Operator1/1 -> Logical Operator/1
  [LstTHState] -> TxtDegraded/2(TxtActv_stLstTHState)
  [TxtLimnum] -> Txt_Tlimit7/2(maxlimit)
  Txt_Tlimit7/1(counter_status) -> [DegradedFlg]
  [THState] -> TxtDegraded/1(TxtActv_stTHState)
  TxtDegraded/1(TxtActv_stDegraded) -> Txt_Tlimit7/1(incrcondition)
  Txt_Tlimit7/2(counter_reset) -> Terminator7/1
  [DegradedFlg] -> Bus Creator1/16  "DegradedFlg"
  [DegradedFlg] -> PrioPrcs/14(DegradedFlg)

== system OMAP_ver_MIL10/OMAP_Module/ICA_Direct_G59/ICA_Define/Subsystem1/Dspl/DsplPrcs/Voc ==
  Voc_stStWhlHld : Inport
  Voc_stTHState : Inport  Port=2
  Voc_dDgrdVocWarnDurnum : Inport  Port=3
  Voc_dHndOffVocWarnnum : Inport  Port=4
  Voc_stVehSty : Inport  Port=5
  Voc_tfAddVocCmd : Inport  Port=6
  Compare To Constant : simulink/Logic and Bit Operations/Compare To Constant  relop===  const=uint16(3)  OutDataTypeStr=boolean
  Compare To Constant1 : simulink/Logic and Bit Operations/Compare To Constant  relop===  const=uint16(4)  OutDataTypeStr=boolean
  Compare To Constant2 : simulink/Logic and Bit Operations/Compare To Constant  relop===  const=uint16(3)  OutDataTypeStr=boolean
  Compare To Constant3 : simulink/Logic and Bit Operations/Compare To Constant  relop===  const=uint16(4)  OutDataTypeStr=boolean
  Compare To Zero1 : simulink/Logic and Bit Operations/Compare To Zero  relop===  OutDataTypeStr=boolean
  Compare To Zero2 : simulink/Logic and Bit Operations/Compare To Zero  relop===  OutDataTypeStr=boolean
  Data Type Conversion{,1..3} (4 alike) : DataTypeConversion  OutDataTypeStr=uint16
  Logical Operator : Logic  AllPortsSameDT=off  OutDataTypeStr=boolean
  Logical Operator1 : Logic  Inputs=3  AllPortsSameDT=off  OutDataTypeStr=boolean
  Logical Operator2 : Logic  Operator=OR  AllPortsSameDT=off  OutDataTypeStr=boolean
  Logical Operator3 : Logic  Operator=OR  AllPortsSameDT=off  OutDataTypeStr=boolean
  MATLAB_Function : MATLAB Function  TreatAsAtomicUnit=on
  Sum_Condition : Subsystem  TreatAsAtomicUnit=on
  Switch : Switch  Criteria=u2 ~= 0
  Unit Delay : UnitDelay  SampleTime=-1
  Voc_stVocDspl : Outport
  wires:
  Voc_stTHState/1 -> Compare To Constant3/1, Compare To Constant2/1, Unit Delay/1, Compare To Constant1/1
  Unit Delay/1 -> Compare To Constant/1
  Compare To Constant1/1 -> Logical Operator/1
  Compare To Constant/1 -> Logical Operator/2
  Logical Operator/1 -> Logical Operator2/1
  Data Type Conversion/1 -> MATLAB_Function/1(Warning_duration)
  Data Type Conversion1/1 -> MATLAB_Function/2(Trigger)
  MATLAB_Function/1(Warning) -> Switch/2, Switch/1
  Voc_stStWhlHld/1 -> Compare To Zero1/1
  Switch/1 -> Voc_stVocDspl/1
  Sum_Condition/1(Out) -> Switch/3
  Data Type Conversion3/1 -> Sum_Condition/Enable, Sum_Condition/1(In)
  Voc_dHndOffVocWarnnum/1 -> Data Type Conversion2/1
  Data Type Conversion2/1 -> Sum_Condition/2(Sum)
  Compare To Zero1/1 -> Logical Operator1/2
  Logical Operator1/1 -> Data Type Conversion3/1
  Voc_dDgrdVocWarnDurnum/1 -> Data Type Conversion/1
  Voc_stVehSty/1 -> Compare To Zero2/1
  Compare To Zero2/1 -> Logical Operator1/3
  Voc_tfAddVocCmd/1 -> Logical Operator2/2
  Logical Operator2/1 -> Data Type Conversion1/1
  Compare To Constant2/1 -> Logical Operator3/1
  Compare To Constant3/1 -> Logical Operator3/2
  Logical Operator3/1 -> Logical Operator1/1

== system OMAP_ver_MIL10/OMAP_Module/ICA_Direct_G59/ICA_Define/Subsystem1/Dspl/DsplPrcs/Icon/FaultInhib ==
  FaultInhib_stTHState : Inport
  FaultInhib_stLstTHState : Inport  Port=2
  FaultInhib_stACCState : Inport  Port=3
  Compare To Constant : simulink/Logic and Bit Operations/Compare To Constant  relop===  const=uint16(15)  OutDataTypeStr=uint8
  Constant : Constant  Value=0  OutDataTypeStr=uint16
  Manual Switch : ManualSwitch  CurrentSetting=0
  FaultInhib_stFaultInhibFlg : Outport
  wires:
  FaultInhib_stACCState/1 -> Compare To Constant/1
  Compare To Constant/1 -> Manual Switch/1
  Constant/1 -> Manual Switch/2
  Manual Switch/1 -> FaultInhib_stFaultInhibFlg/1

== system OMAP_ver_MIL10/OMAP_Module/ICA_Direct_G59/ICA_Define/Subsystem1/Dspl/DsplPrcs/Icon/else ==
  HiDurnum : Inport
  LoDurnum : Inport  Port=2
  Action Port : ActionPort  InitializeStates=reset
  Add : Sum
  Constant1 : Constant  Value=0  OutDataTypeStr=uint16
  Constant8 : Constant  OutDataTypeStr=uint16
  Relational Operator1 : RelationalOperator  Operator=<=  OutDataTypeStr=boolean  RndMeth=Nearest
  Relational Operator2 : RelationalOperator  Operator=<=  OutDataTypeStr=boolean  RndMeth=Nearest
  Sum : Sum  OutDataTypeStr=Inherit: Inherit via back propagation  InputSameDT=on
  Unit Delay1 : UnitDelay  SampleTime=-1
  Unit Delay2 : UnitDelay  SampleTime=-1
  reset switch1 : Switch  Criteria=u2 ~= 0  Threshold=1  OutDataTypeStr=Inherit: Inherit via back propagation  InputSameDT=on
  count : Outport
  counter_status : Outport  Port=2
  wires:
  Unit Delay2/1 -> Sum/2
  Constant8/1 -> Sum/1
  Sum/1 -> reset switch1/3
  [reset] -> reset switch1/2
  Constant1/1 -> reset switch1/1
  Relational Operator1/1 -> Unit Delay1/1
  Unit Delay1/1 -> [reset]
  reset switch1/1 -> Unit Delay2/1, Relational Operator1/2, Relational Operator2/1, count/1
  Relational Operator2/1 -> counter_status/1
  Add/1 -> Relational Operator1/1
  LoDurnum/1 -> Add/2
  HiDurnum/1 -> Add/1, Relational Operator2/2

== system OMAP_ver_MIL10/OMAP_Module/ICA_Direct_G59/ICA_Define/Subsystem1/Dspl/DsplPrcs/Icon/gray ==
  In1 : Inport
  Action Port : ActionPort
  Out1 : Outport
  wires:
  In1/1 -> Out1/1

== system OMAP_ver_MIL10/OMAP_Module/ICA_Direct_G59/ICA_Define/Subsystem1/Dspl/DsplPrcs/Icon/green ==
  In1 : Inport
  Action Port : ActionPort
  Out1 : Outport
  wires:
  In1/1 -> Out1/1

== system OMAP_ver_MIL10/OMAP_Module/ICA_Direct_G59/ICA_Define/Subsystem1/Dspl/DsplPrcs/Icon/hold_last ==
  In1 : Inport
  Action Port : ActionPort
  Out1 : Outport
  wires:
  In1/1 -> Out1/1

== system OMAP_ver_MIL10/OMAP_Module/ICA_Direct_G59/ICA_Define/Subsystem1/Dspl/DsplPrcs/Icon/if ==
  In1 : Inport
  Action Port : ActionPort
  Out1 : Outport
  wires:
  In1/1 -> Out1/1

== system OMAP_ver_MIL10/OMAP_Module/ICA_Direct_G59/ICA_Define/Subsystem1/Dspl/DsplPrcs/Icon/off ==
  In1 : Inport
  Action Port : ActionPort
  Out1 : Outport
  wires:
  In1/1 -> Out1/1

== system OMAP_ver_MIL10/OMAP_Module/ICA_Direct_G59/ICA_Define/Subsystem1/Dspl/DsplPrcs/Icon/off_fault ==
  In1 : Inport
  Action Port : ActionPort
  Out1 : Outport
  wires:
  In1/1 -> Out1/1

== system OMAP_ver_MIL10/OMAP_Module/ICA_Direct_G59/ICA_Define/Subsystem1/Dspl/DsplPrcs/Icon/orange ==
  In1 : Inport
  In2 : Inport  Port=2
  Action Port : ActionPort
  Compare To Constant : simulink/Logic and Bit Operations/Compare To Constant  relop===  const=boolean(1)  OutDataTypeStr=boolean
  Constant7 : Constant  Value=0  OutDataTypeStr=uint16
  reset switch1 : Switch  Criteria=u2 ~= 0  Threshold=1  OutDataTypeStr=Inherit: Inherit via back propagation  InputSameDT=on
  Out1 : Outport
  wires:
  Compare To Constant/1 -> reset switch1/2
  reset switch1/1 -> Out1/1
  Constant7/1 -> reset switch1/3
  In2/1 -> Compare To Constant/1
  In1/1 -> reset switch1/1

== system OMAP_ver_MIL10/OMAP_Module/ICA_Direct_G59/ICA_Define/Subsystem1/Dspl/DsplPrcs/Icon/red ==
  In1 : Inport
  Action Port : ActionPort
  Out1 : Outport
  wires:
  In1/1 -> Out1/1

== system OMAP_ver_MIL10/OMAP_Module/ICA_Direct_G59/ICA_Define/Subsystem1/Dspl/DsplPrcs/Lane/Subsystem ==
  In1 : Inport
  Enable : EnablePort
  Out1 : Outport
  wires:
  In1/1 -> Out1/1

== system OMAP_ver_MIL10/OMAP_Module/ICA_Direct_G59/ICA_Define/Subsystem1/Dspl/DsplPrcs/Lane/left_no_right_no ==
  In1 : Inport
  In2 : Inport  Port=2
  In3 : Inport  Port=3
  Action Port : ActionPort
  Out1 : Outport
  Out2 : Outport  Port=2
  Out3 : Outport  Port=3
  wires:
  In1/1 -> Out1/1
  In2/1 -> Out2/1
  In3/1 -> Out3/1

== system OMAP_ver_MIL10/OMAP_Module/ICA_Direct_G59/ICA_Define/Subsystem1/Dspl/DsplPrcs/Lane/left_no_right_no1 ==
  In1 : Inport
  In2 : Inport  Port=2
  In3 : Inport  Port=3
  Action Port : ActionPort
  Out1 : Outport
  Out2 : Outport  Port=2
  Out3 : Outport  Port=3
  wires:
  In3/1 -> Out3/1
  In2/1 -> Out2/1
  In1/1 -> Out1/1

== system OMAP_ver_MIL10/OMAP_Module/ICA_Direct_G59/ICA_Define/Subsystem1/Dspl/DsplPrcs/Lane/left_no_right_ok ==
  In1 : Inport
  In2 : Inport  Port=2
  In3 : Inport  Port=3
  Action Port : ActionPort
  Out1 : Outport
  Out2 : Outport  Port=2
  Out3 : Outport  Port=3
  wires:
  In3/1 -> Out3/1
  In2/1 -> Out2/1
  In1/1 -> Out1/1

== system OMAP_ver_MIL10/OMAP_Module/ICA_Direct_G59/ICA_Define/Subsystem1/Dspl/DsplPrcs/Lane/left_ok_right_no ==
  In1 : Inport
  In2 : Inport  Port=2
  In3 : Inport  Port=3
  Action Port : ActionPort
  Out1 : Outport
  Out2 : Outport  Port=2
  Out3 : Outport  Port=3
  wires:
  In1/1 -> Out1/1
  In2/1 -> Out2/1
  In3/1 -> Out3/1

== system OMAP_ver_MIL10/OMAP_Module/ICA_Direct_G59/ICA_Define/Subsystem1/Dspl/DsplPrcs/Lane/left_ok_right_ok ==
  In1 : Inport
  In2 : Inport  Port=2
  In3 : Inport  Port=3
  Action Port : ActionPort
  Out1 : Outport
  Out2 : Outport  Port=2
  Out3 : Outport  Port=3
  wires:
  In3/1 -> Out3/1
  In2/1 -> Out2/1
  In1/1 -> Out1/1

== system OMAP_ver_MIL10/OMAP_Module/ICA_Direct_G59/ICA_Define/Subsystem1/Dspl/DsplPrcs/Lane_old/Subsystem ==
  In1 : Inport
  Enable : EnablePort
  Out1 : Outport
  wires:
  In1/1 -> Out1/1

== system OMAP_ver_MIL10/OMAP_Module/ICA_Direct_G59/ICA_Define/Subsystem1/Dspl/DsplPrcs/Lane_old/both_gray ==
  In1 : Inport
  Action Port : ActionPort
  Out1 : Outport
  wires:
  In1/1 -> Out1/1

== system OMAP_ver_MIL10/OMAP_Module/ICA_Direct_G59/ICA_Define/Subsystem1/Dspl/DsplPrcs/Lane_old/both_green ==
  In1 : Inport
  Action Port : ActionPort
  Out1 : Outport
  wires:
  In1/1 -> Out1/1

== system OMAP_ver_MIL10/OMAP_Module/ICA_Direct_G59/ICA_Define/Subsystem1/Dspl/DsplPrcs/Lane_old/left_green ==
  In1 : Inport
  Action Port : ActionPort
  Out1 : Outport
  wires:
  In1/1 -> Out1/1

== system OMAP_ver_MIL10/OMAP_Module/ICA_Direct_G59/ICA_Define/Subsystem1/Dspl/DsplPrcs/Lane_old/no_lane ==
  In1 : Inport
  Action Port : ActionPort
  Out1 : Outport
  wires:
  In1/1 -> Out1/1

== system OMAP_ver_MIL10/OMAP_Module/ICA_Direct_G59/ICA_Define/Subsystem1/Dspl/DsplPrcs/Lane_old/right_green ==
  In1 : Inport
  Action Port : ActionPort
  Out1 : Outport
  wires:
  In1/1 -> Out1/1

== system OMAP_ver_MIL10/OMAP_Module/ICA_Direct_G59/ICA_Define/Subsystem1/Dspl/DsplPrcs/Txt/HndOffTxtTlimit ==
  incrcondition : Inport
  reset : Inport  Port=2
  maxlimit : Inport  Port=3
  Constant : Constant  Value=0  OutDataTypeStr=uint16
  Constant1 : Constant  OutDataTypeStr=uint16
  Constant2 : Constant  Value=0  OutDataTypeStr=uint16
  Constant3 : Constant  Value=0  OutDataTypeStr=uint16
  MinMax1 : MinMax  Inputs=2  OutDataTypeStr=Inherit: Inherit via back propagation  InputSameDT=on
  MinMax2 : MinMax  Function=max  Inputs=2  OutDataTypeStr=Inherit: Inherit via back propagation  InputSameDT=on
  Relational Operator : RelationalOperator  OutDataTypeStr=boolean  RndMeth=Nearest
  Sum : Sum  OutDataTypeStr=Inherit: Inherit via back propagation  InputSameDT=on
  Unit Delay : UnitDelay  SampleTime=-1
  inc switch : Switch  Criteria=u2 ~= 0  Threshold=1  OutDataTypeStr=Inherit: Inherit via back propagation  InputSameDT=on
  reset switch : Switch  Criteria=u2 ~= 0  Threshold=1  OutDataTypeStr=Inherit: Inherit via back propagation  InputSameDT=on
  counter_out : Outport
  counter_status : Outport  Port=2
  wires:
  Relational Operator/1 -> counter_status/1
  reset switch/1 -> counter_out/1, Unit Delay/1, Relational Operator/1
  Constant2/1 -> MinMax2/1
  incrcondition/1 -> inc switch/2
  maxlimit/1 -> Relational Operator/2, MinMax1/2
  MinMax2/1 -> MinMax1/1
  Constant/1 -> inc switch/3
  Constant1/1 -> inc switch/1
  MinMax1/1 -> reset switch/3
  reset/1 -> reset switch/2
  Sum/1 -> MinMax2/2
  inc switch/1 -> Sum/2
  Constant3/1 -> reset switch/1
  Unit Delay/1 -> Sum/1

== system OMAP_ver_MIL10/OMAP_Module/ICA_Direct_G59/ICA_Define/Subsystem1/Dspl/DsplPrcs/Txt/TxtActv ==
  TxtActv_stTHState : Inport
  TxtActv_stLstTHState : Inport  Port=2
  Constant1 : Constant  OutDataTypeStr=uint16
  Constant2 : Constant  Value=0  OutDataTypeStr=uint16
  Hold : Subsystem  TreatAsAtomicUnit=on
  If : If  NumInputs=2  IfExpression=(u1 == 3 |u1 == 4 |u1 == 6) & u2 == 2  ElseIfExpressions=u1 ~= 3 & u1 ~= 4 & u1 ~= 6
  Merge : Merge  Inputs=3
  Start : Subsystem  TreatAsAtomicUnit=on
  Stop : Subsystem  TreatAsAtomicUnit=on
  Unit Delay1 : UnitDelay  SampleTime=-1
  TxtActv_stActv : Outport
  wires:
  TxtActv_stTHState/1 -> If/1
  Merge/1 -> Unit Delay1/1, TxtActv_stActv/1
  Start/1(Out1) -> Merge/1
  TxtActv_stLstTHState/1 -> If/2
  Constant1/1 -> Start/1(In1)
  If/1 -> Start/Action
  Constant2/1 -> Stop/1(In1)
  If/2 -> Stop/Action
  Unit Delay1/1 -> Hold/1(In1)
  If/3 -> Hold/Action
  Stop/1(Out1) -> Merge/2
  Hold/1(Out1) -> Merge/3

== system OMAP_ver_MIL10/OMAP_Module/ICA_Direct_G59/ICA_Define/Subsystem1/Dspl/DsplPrcs/Txt/TxtCncl ==
  TxtCncl_stTHState : Inport
  TxtCncl_stLstTHState : Inport  Port=2
  Constant1 : Constant  OutDataTypeStr=uint16
  Constant2 : Constant  Value=0  OutDataTypeStr=uint16
  Hold : Subsystem  TreatAsAtomicUnit=on
  If : If  NumInputs=2  IfExpression=u1 == 1 & (u2 == 3 | u2 == 4 | u2 == 6)  ElseIfExpressions=u1 ~= 1 & u1 ~= 2
  Merge : Merge  Inputs=3
  Start : Subsystem  TreatAsAtomicUnit=on
  Stop : Subsystem  TreatAsAtomicUnit=on
  Unit Delay1 : UnitDelay  SampleTime=-1
  TxtCncl_stCncl : Outport
  wires:
  Hold/1(Out1) -> Merge/3
  Stop/1(Out1) -> Merge/2
  If/3 -> Hold/Action
  Unit Delay1/1 -> Hold/1(In1)
  If/2 -> Stop/Action
  Constant2/1 -> Stop/1(In1)
  If/1 -> Start/Action
  Constant1/1 -> Start/1(In1)
  TxtCncl_stLstTHState/1 -> If/2
  Start/1(Out1) -> Merge/1
  Merge/1 -> TxtCncl_stCncl/1, Unit Delay1/1
  TxtCncl_stTHState/1 -> If/1

== system OMAP_ver_MIL10/OMAP_Module/ICA_Direct_G59/ICA_Define/Subsystem1/Dspl/DsplPrcs/Txt/TxtDegraded ==
  TxtActv_stTHState : Inport
  TxtActv_stLstTHState : Inport  Port=2
  Constant1 : Constant  OutDataTypeStr=uint16
  Constant2 : Constant  Value=0  OutDataTypeStr=uint16
  Hold : Subsystem  TreatAsAtomicUnit=on
  If : If  NumInputs=2  IfExpression=u1 == 4 & u2 == 4  ElseIfExpressions=u1 ~= 4 & u2 == 4
  Merge : Merge  Inputs=3
  Start : Subsystem  TreatAsAtomicUnit=on
  Stop : Subsystem  TreatAsAtomicUnit=on
  Unit Delay1 : UnitDelay  SampleTime=-1
  TxtActv_stDegraded : Outport
  wires:
  TxtActv_stTHState/1 -> If/1
  Merge/1 -> Unit Delay1/1, TxtActv_stDegraded/1
  Start/1(Out1) -> Merge/1
  TxtActv_stLstTHState/1 -> If/2
  Constant1/1 -> Start/1(In1)
  If/1 -> Start/Action
  Constant2/1 -> Stop/1(In1)
  If/2 -> Stop/Action
  Unit Delay1/1 -> Hold/1(In1)
  If/3 -> Hold/Action
  Stop/1(Out1) -> Merge/2
  Hold/1(Out1) -> Merge/3

== system OMAP_ver_MIL10/OMAP_Module/ICA_Direct_G59/ICA_Define/Subsystem1/Dspl/DsplPrcs/Txt/TxtFromACC ==
  TxtFromACC_stTHState : Inport
  TxtFromACC_stLstTHState : Inport  Port=2
  TxtFromACC_stACCTxtDspl : Inport  Port=3
  TxtFromACC_stSWALimFlg : Inport  Port=4
  TxtFromACC_tiSWALimFlgDetnum : Inport  Port=5
  TxtFromACC_stTkOvStChk : Inport  Port=6
  Compare To Constant : simulink/Logic and Bit Operations/Compare To Constant  relop===  const=uint16(3)  OutDataTypeStr=boolean
  Constant{1,3,5,7,9} (5 alike) : Constant  OutDataTypeStr=uint16
  Constant{2,4,6,8,10} (5 alike) : Constant  Value=0  OutDataTypeStr=uint16
  Data Type Conversion14 : DataTypeConversion  OutDataTypeStr=uint16
  Data Type Conversion2 : DataTypeConversion  OutDataTypeStr=uint16
  Enabled Subsystem : Subsystem  TreatAsAtomicUnit=on
  Hold : Subsystem  TreatAsAtomicUnit=on
  If : If  NumInputs=2  IfExpression=( u1 == 3 |u1 == 4 |u1 == 6 )& u2 == 6
  If1 : If  NumInputs=2  IfExpression=( u1 == 3 |u1 == 4 |u1 == 6 )& u2 == 7
  If2 : If  NumInputs=2  IfExpression=( u1 == 3 |u1 == 4 |u1 == 6 )& u2 == 8
  If3 : If  NumInputs=3  IfExpression=u1 == 5 & u2 == 2 & u3 == 0
  If4 : If  NumInputs=2  IfExpression=u1 == 1  ElseIfExpressions=u2 == 1
  Logical Operator : Logic  Operator=OR  AllPortsSameDT=off  OutDataTypeStr=boolean
  Logical Operator1 : Logic  AllPortsSameDT=off  OutDataTypeStr=boolean
  Merge{,1..3} (4 alike) : Merge
  Merge4 : Merge  Inputs=3
  RdrBlkInhib : Subsystem
  Start : Subsystem  TreatAsAtomicUnit=on
  Start1 : Subsystem  TreatAsAtomicUnit=on
  Start2 : Subsystem  TreatAsAtomicUnit=on
  Start3 : Subsystem  TreatAsAtomicUnit=on
  Start4 : Subsystem  TreatAsAtomicUnit=on
  Stop : Subsystem  TreatAsAtomicUnit=on
  Stop1 : Subsystem  TreatAsAtomicUnit=on
  Stop2 : Subsystem  TreatAsAtomicUnit=on
  Stop3 : Subsystem  TreatAsAtomicUnit=on
  Stop4 : Subsystem  TreatAsAtomicUnit=on
  Unit Delay1 : UnitDelay  SampleTime=-1
  TxtFromACC_stGoReq : Outport
  TxtFromACC_stTkOv : Outport  Port=2
  TxtFromACC_stImmdTkOv : Outport  Port=3
  TxtFromACC_stRdrBlk : Outport  Port=4
  wires:
  Stop/1(Out1) -> Merge/2
  Constant2/1 -> Stop/1(In1)
  If/1 -> Start/Action
  Constant1/1 -> Start/1(In1)
  Start/1(Out1) -> Merge/1
  Merge/1 -> TxtFromACC_stGoReq/1
  If/2 -> Stop/Action
  TxtFromACC_stTHState/1 -> [THState]
  If1/2 -> Stop1/Action
  Stop1/1(Out1) -> Merge1/2
  Start1/1(Out1) -> Merge1/1
  Constant4/1 -> Stop1/1(In1)
  If1/1 -> Start1/Action
  Merge1/1 -> TxtFromACC_stTkOv/1
  Constant3/1 -> Start1/1(In1)
  If2/2 -> Stop2/Action
  Stop2/1(Out1) -> Merge2/2
  Start2/1(Out1) -> Merge2/1
  Constant6/1 -> Stop2/1(In1)
  If2/1 -> Start2/Action
  Constant5/1 -> Start2/1(In1)
  TxtFromACC_stLstTHState/1 -> RdrBlkInhib/2(RdrBlkInhib_stLstTHState)
  TxtFromACC_stACCTxtDspl/1 -> [ACCTxtDspl]
  [THState] -> If/1
  [ACCTxtDspl] -> If/2
  [THState] -> If1/1
  [ACCTxtDspl] -> If1/2
  [THState] -> If2/1
  [ACCTxtDspl] -> If2/2
  [THState] -> RdrBlkInhib/1(RdrBlkInhib_stTHState)
  [ACCTxtDspl] -> RdrBlkInhib/3(RdrBlkInhib_stACCTxtDspl)
  If3/2 -> Stop3/Action
  Start3/1(Out1) -> Merge3/1
  If3/1 -> Start3/Action
  Constant7/1 -> Start3/1(In1)
  Constant8/1 -> Stop3/1(In1)
  Stop3/1(Out1) -> Merge3/2
  [ACCTxtDspl] -> If3/2
  [THState] -> If3/1
  Merge3/1 -> TxtFromACC_stRdrBlk/1
  RdrBlkInhib/1(RdrBlkInhib_stRdrBlkInhibFlg) -> If3/3
  TxtFromACC_stSWALimFlg/1 -> Logical Operator1/2
  TxtFromACC_stTkOvStChk/1 -> If4/2
  If4/2 -> Stop4/Action
  Stop4/1(Out1) -> Merge4/2
  Start4/1(Out1) -> Merge4/1
  Constant10/1 -> Stop4/1(In1)
  If4/1 -> Start4/Action
  Constant9/1 -> Start4/1(In1)
  Hold/1(Out1) -> Merge4/3
  Unit Delay1/1 -> Hold/1(In1)
  Merge4/1 -> Logical Operator/2, Unit Delay1/1
  If4/3 -> Hold/Action
  Merge2/1 -> Logical Operator/1
  Logical Operator/1 -> Data Type Conversion14/1
  Data Type Conversion14/1 -> TxtFromACC_stImmdTkOv/1
  [THState] -> Compare To Constant/1
  Compare To Constant/1 -> Logical Operator1/1
  Data Type Conversion2/1 -> If4/1
  TxtFromACC_tiSWALimFlgDetnum/1 -> Enabled Subsystem/1(Num)
  Enabled Subsystem/1(Triger) -> Data Type Conversion2/1
  Logical Operator1/1 -> Enabled Subsystem/Enable

== system OMAP_ver_MIL10/OMAP_Module/ICA_Direct_G59/ICA_Define/Subsystem1/Dspl/DsplPrcs/Txt/TxtInactv ==
  TxtInactv_stTHState : Inport
  TxtInactv_stTHFKeyState : Inport  Port=2
  TxtInactv_stCntRst : Inport  Port=3
  Constant1 : Constant  OutDataTypeStr=uint16
  Constant2 : Constant  Value=0  OutDataTypeStr=uint16
  Hold : Subsystem  TreatAsAtomicUnit=on
  If : If  NumInputs=3  IfExpression=u1 ~= 1 | u3 == 1  ElseIfExpressions=u1 == 1 & (u2 == 3 | u2 == 4)
  Merge : Merge  Inputs=3
  Start : Subsystem  TreatAsAtomicUnit=on
  Stop : Subsystem  TreatAsAtomicUnit=on
  Unit Delay1 : UnitDelay  SampleTime=-1
  TxtInactv_stInactv : Outport
  wires:
  Hold/1(Out1) -> Merge/3
  Start/1(Out1) -> Merge/2
  If/3 -> Hold/Action
  Unit Delay1/1 -> Hold/1(In1)
  If/2 -> Start/Action
  If/1 -> Stop/Action
  TxtInactv_stTHFKeyState/1 -> If/2
  Stop/1(Out1) -> Merge/1
  Merge/1 -> TxtInactv_stInactv/1, Unit Delay1/1
  TxtInactv_stTHState/1 -> If/1
  TxtInactv_stCntRst/1 -> If/3
  Constant1/1 -> Start/1(In1)
  Constant2/1 -> Stop/1(In1)
